simulink model "test_1"  (R2019b)
settings: Solver=VariableStepAuto  StartTime=0.0  StopTime=Tend  RelTol=1e-3
values from neighbouring files (symbols this model uses):
  den = [1 1]    [tset_1.m]
  num = [1]    [tset_1.m]
  Tend = 40    [tset_1.m]
  w1 = fmax*2*pi    (= 0.948760981384)    [tset_1.m]
libraries: simulink x1
settings Model: Creator=朱佳琪  LastModifiedBy=朱佳琪

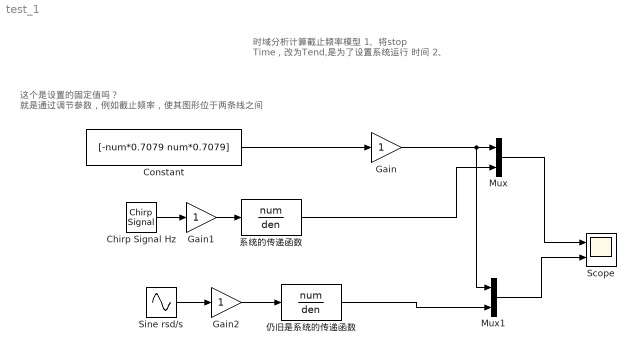
== system test_1 ==
  note: 这个是设置的固定值吗？
      | 就是通过调节参数，例如截止频率，使其图形位于两条线之间
  note: 时域分析计算截止频率模型
      | 1、将stop Time，改为Tend,是为了设置系统运行 时间
      | 2、
  " 仍旧是系统的传递函数" : TransferFcn  Numerator=num  Denominator=den
  Chirp Signal Hz : simulink/Sources/Chirp Signal  f1=Fstart  T=Tend  f2=Fend
  Constant : Constant  Value=[-num*0.7079 num*0.7079]
  Gain : Gain
  Gain1 : Gain
  Gain2 : Gain
  Mux : Mux  Inputs=2
  Mux1 : Mux  Inputs=2
  Scope : Scope  NumInputPorts=2
  Sine rsd/s : Sin  Frequency=w1  SampleTime=0
  系统的传递函数 : TransferFcn  Numerator=num  Denominator=den
  wires:
  Sine rsd/s/1 -> Gain2/1
  Chirp Signal Hz/1 -> Gain1/1
  Constant/1 -> Gain/1
  Gain/1 -> Mux1/1, Mux/1
  系统的传递函数/1 -> Mux/2
  Mux/1 -> Scope/1
  " 仍旧是系统的传递函数"/1 -> Mux1/2
  Mux1/1 -> Scope/2
  Gain1/1 -> 系统的传递函数/1
  Gain2/1 -> " 仍旧是系统的传递函数"/1
